simulink library "Completemodels"  (R2014b)
settings: Solver=ode45  StartTime=0.0  StopTime=10.0  RelTol=1e-3
undefined symbols (not defined in the file): X, Y, Z
libraries: sm_lib x26, nesl_utility x24, HexapodLib x18, ServoModel x18, simulink x2
settings Model: Creator=Sebastian  LastModifiedBy=Sebastian

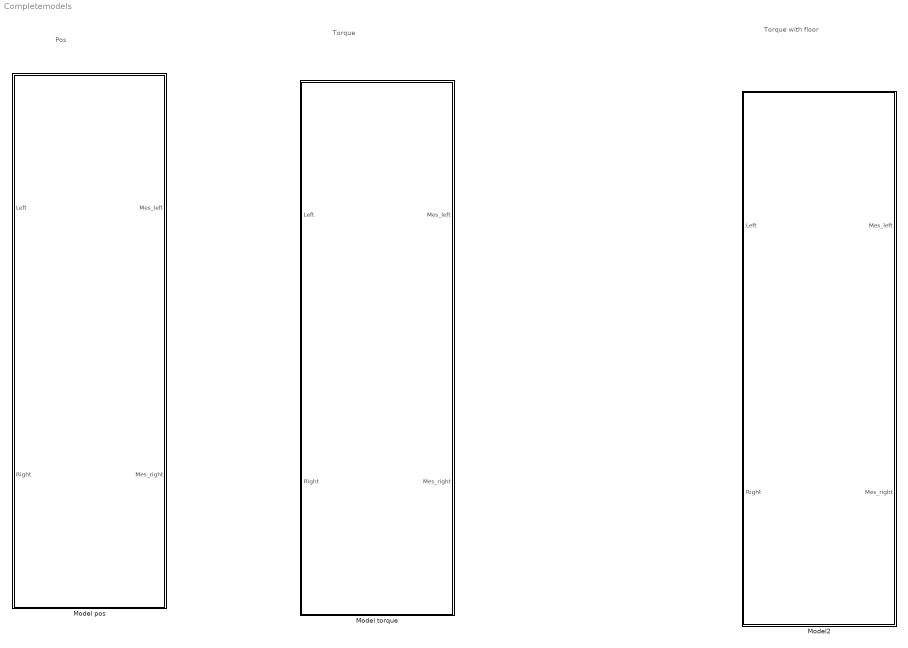
== system Completemodels ==
  note: Pos
  note: Torque
  note: Torque with floor
  Model pos : Subsystem
  Model torque : Subsystem
  Model2 : Subsystem

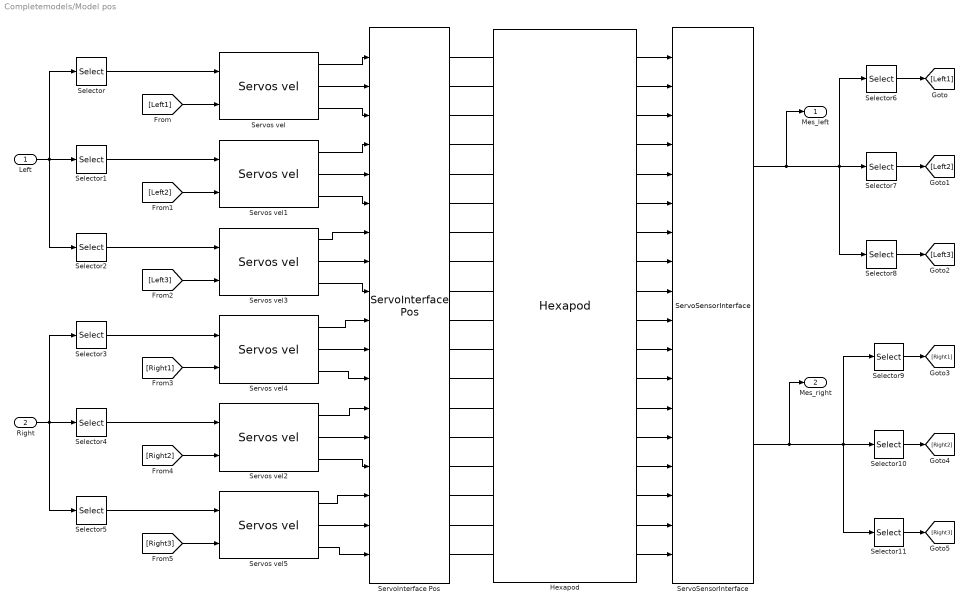
== system Completemodels/Model pos ==
  Left : Inport
  Right : Inport  Port=2
  Hexapod : HexapodLib/Hexapod
  Selector{,3,6,9} (4 alike) : Selector  IndexMode=Zero-based  InputPortWidth=3  Indices=0
  Selector{1,4,7,10} (4 alike) : Selector  IndexMode=Zero-based  InputPortWidth=3
  Selector{2,5,8,11} (4 alike) : Selector  IndexMode=Zero-based  InputPortWidth=3  Indices=2
  ServoInterface Pos : HexapodLib/ServoInterface Pos  Filter_time=0.001
  ServoSensorInterface : HexapodLib/ServoSensorInterface
  Servos vel{,1..5} (6 alike) : ServoModel/Servos vel
  Mes_left : Outport
  Mes_right : Outport  Port=2
  wires:
  Hexapod/9 -> ServoSensorInterface/9
  Servos vel1/1 -> ServoInterface Pos/4
  Hexapod/5 -> ServoSensorInterface/5
  Servos vel5/1 -> ServoInterface Pos/16
  [Right3] -> Servos vel5/2
  Servos vel4/1 -> ServoInterface Pos/10
  Servos vel3/2 -> ServoInterface Pos/8
  Servos vel/2 -> ServoInterface Pos/2
  Servos vel2/3 -> ServoInterface Pos/15
  [Left1] -> Servos vel/2
  [Right1] -> Servos vel4/2
  Servos vel/1 -> ServoInterface Pos/1
  Servos vel/3 -> ServoInterface Pos/3
  Servos vel4/3 -> ServoInterface Pos/12
  Servos vel2/2 -> ServoInterface Pos/14
  [Left3] -> Servos vel3/2
  Servos vel1/3 -> ServoInterface Pos/6
  Servos vel5/3 -> ServoInterface Pos/18
  Servos vel1/2 -> ServoInterface Pos/5
  [Right2] -> Servos vel2/2
  Servos vel3/3 -> ServoInterface Pos/9
  Servos vel4/2 -> ServoInterface Pos/11
  [Left2] -> Servos vel1/2
  Servos vel2/1 -> ServoInterface Pos/13
  Servos vel3/1 -> ServoInterface Pos/7
  Hexapod/10 -> ServoSensorInterface/10
  Hexapod/7 -> ServoSensorInterface/7
  Hexapod/4 -> ServoSensorInterface/4
  Servos vel5/2 -> ServoInterface Pos/17
  Hexapod/8 -> ServoSensorInterface/8
  Hexapod/3 -> ServoSensorInterface/3
  Hexapod/2 -> ServoSensorInterface/2
  Hexapod/1 -> ServoSensorInterface/1
  Hexapod/6 -> ServoSensorInterface/6
  Hexapod/18 -> ServoSensorInterface/18
  Hexapod/17 -> ServoSensorInterface/17
  Hexapod/16 -> ServoSensorInterface/16
  Hexapod/15 -> ServoSensorInterface/15
  Hexapod/14 -> ServoSensorInterface/14
  Hexapod/13 -> ServoSensorInterface/13
  Hexapod/12 -> ServoSensorInterface/12
  Hexapod/11 -> ServoSensorInterface/11
  Left/1 -> Selector2/1, Selector/1, Selector1/1
  Selector1/1 -> Servos vel1/1
  Selector/1 -> Servos vel/1
  Selector2/1 -> Servos vel3/1
  Right/1 -> Selector3/1, Selector5/1, Selector4/1
  Selector4/1 -> Servos vel2/1
  Selector3/1 -> Servos vel4/1
  Selector5/1 -> Servos vel5/1
  ServoSensorInterface/1 -> Selector8/1, Selector6/1, Selector7/1, Mes_left/1
  Selector6/1 -> [Left1]
  Selector7/1 -> [Left2]
  Selector8/1 -> [Left3]
  ServoSensorInterface/2 -> Selector11/1, Selector9/1, Selector10/1, Mes_right/1
  Selector9/1 -> [Right1]
  Selector10/1 -> [Right2]
  Selector11/1 -> [Right3]
  connections:
  Hexapod/LConn7 -- ServoInterface Pos/RConn7
  Hexapod/LConn5 -- ServoInterface Pos/RConn5
  Hexapod/LConn3 -- ServoInterface Pos/RConn3
  Hexapod/LConn16 -- ServoInterface Pos/RConn16
  Hexapod/LConn15 -- ServoInterface Pos/RConn15
  Hexapod/LConn18 -- ServoInterface Pos/RConn18
  Hexapod/LConn14 -- ServoInterface Pos/RConn14
  Hexapod/LConn13 -- ServoInterface Pos/RConn13
  Hexapod/LConn17 -- ServoInterface Pos/RConn17
  Hexapod/LConn11 -- ServoInterface Pos/RConn11
  Hexapod/LConn12 -- ServoInterface Pos/RConn12
  Hexapod/LConn10 -- ServoInterface Pos/RConn10
  Hexapod/LConn8 -- ServoInterface Pos/RConn8
  Hexapod/LConn9 -- ServoInterface Pos/RConn9
  Hexapod/LConn2 -- ServoInterface Pos/RConn2
  Hexapod/LConn4 -- ServoInterface Pos/RConn4
  Hexapod/LConn6 -- ServoInterface Pos/RConn6
  Hexapod/LConn1 -- ServoInterface Pos/RConn1

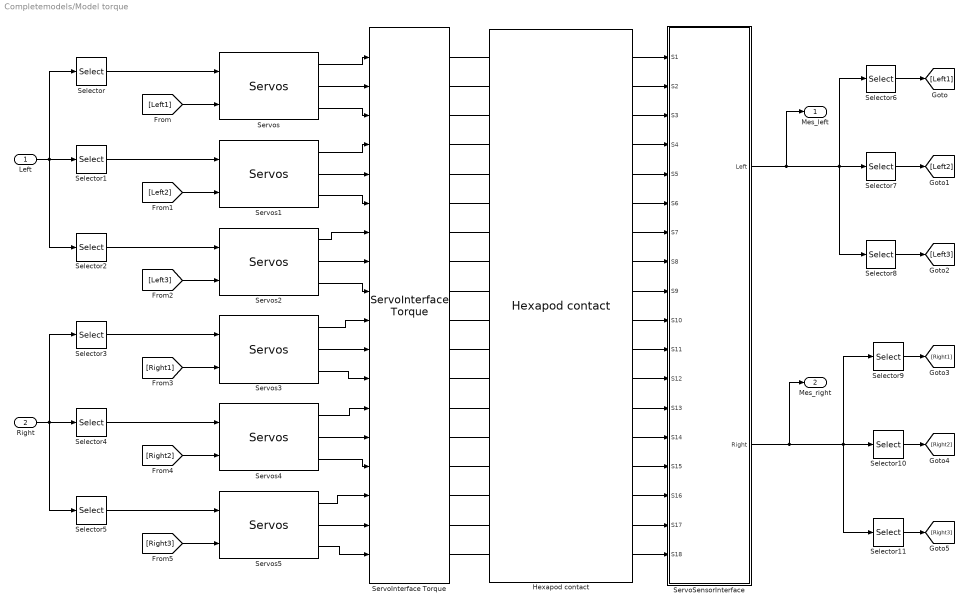
== system Completemodels/Model torque ==
  Left : Inport
  Right : Inport  Port=2
  Hexapod contact : HexapodLib/Hexapod contact
  Selector{,3,6,9} (4 alike) : Selector  IndexMode=Zero-based  InputPortWidth=3  Indices=0
  Selector{1,4,7,10} (4 alike) : Selector  IndexMode=Zero-based  InputPortWidth=3
  Selector{2,5,8,11} (4 alike) : Selector  IndexMode=Zero-based  InputPortWidth=3  Indices=2
  ServoInterface Torque : HexapodLib/ServoInterface Torque
  ServoSensorInterface : Subsystem
  Servos{,1..5} (6 alike) : ServoModel/Servos
  Mes_left : Outport
  Mes_right : Outport  Port=2
  wires:
  Hexapod contact/9 -> ServoSensorInterface/9(S9)
  Servos1/1 -> ServoInterface Torque/4
  Hexapod contact/5 -> ServoSensorInterface/5(S5)
  Servos5/1 -> ServoInterface Torque/16
  [Right3] -> Servos5/2
  Servos3/1 -> ServoInterface Torque/10
  Servos2/2 -> ServoInterface Torque/8
  Servos/2 -> ServoInterface Torque/2
  Servos4/3 -> ServoInterface Torque/15
  [Left1] -> Servos/2
  [Right1] -> Servos3/2
  Servos/1 -> ServoInterface Torque/1
  Servos/3 -> ServoInterface Torque/3
  Servos3/3 -> ServoInterface Torque/12
  Servos4/2 -> ServoInterface Torque/14
  [Left3] -> Servos2/2
  Servos1/3 -> ServoInterface Torque/6
  Servos5/3 -> ServoInterface Torque/18
  Servos1/2 -> ServoInterface Torque/5
  [Right2] -> Servos4/2
  Servos2/3 -> ServoInterface Torque/9
  Servos3/2 -> ServoInterface Torque/11
  [Left2] -> Servos1/2
  Servos4/1 -> ServoInterface Torque/13
  Servos2/1 -> ServoInterface Torque/7
  Hexapod contact/10 -> ServoSensorInterface/10(S10)
  Hexapod contact/7 -> ServoSensorInterface/7(S7)
  Hexapod contact/4 -> ServoSensorInterface/4(S4)
  Servos5/2 -> ServoInterface Torque/17
  Hexapod contact/8 -> ServoSensorInterface/8(S8)
  Hexapod contact/3 -> ServoSensorInterface/3(S3)
  Hexapod contact/2 -> ServoSensorInterface/2(S2)
  Hexapod contact/1 -> ServoSensorInterface/1(S1)
  Hexapod contact/6 -> ServoSensorInterface/6(S6)
  Hexapod contact/18 -> ServoSensorInterface/18(S18)
  Hexapod contact/17 -> ServoSensorInterface/17(S17)
  Hexapod contact/16 -> ServoSensorInterface/16(S16)
  Hexapod contact/15 -> ServoSensorInterface/15(S15)
  Hexapod contact/14 -> ServoSensorInterface/14(S14)
  Hexapod contact/13 -> ServoSensorInterface/13(S13)
  Hexapod contact/12 -> ServoSensorInterface/12(S12)
  Hexapod contact/11 -> ServoSensorInterface/11(S11)
  Left/1 -> Selector2/1, Selector/1, Selector1/1
  Selector1/1 -> Servos1/1
  Selector/1 -> Servos/1
  Selector2/1 -> Servos2/1
  Right/1 -> Selector3/1, Selector5/1, Selector4/1
  Selector4/1 -> Servos4/1
  Selector3/1 -> Servos3/1
  Selector5/1 -> Servos5/1
  ServoSensorInterface/1(Left) -> Selector8/1, Selector6/1, Selector7/1, Mes_left/1
  Selector6/1 -> [Left1]
  Selector7/1 -> [Left2]
  Selector8/1 -> [Left3]
  ServoSensorInterface/2(Right) -> Selector11/1, Selector9/1, Selector10/1, Mes_right/1
  Selector9/1 -> [Right1]
  Selector10/1 -> [Right2]
  Selector11/1 -> [Right3]
  connections:
  Hexapod contact/LConn7 -- ServoInterface Torque/RConn7
  Hexapod contact/LConn5 -- ServoInterface Torque/RConn5
  Hexapod contact/LConn3 -- ServoInterface Torque/RConn3
  Hexapod contact/LConn16 -- ServoInterface Torque/RConn16
  Hexapod contact/LConn15 -- ServoInterface Torque/RConn15
  Hexapod contact/LConn18 -- ServoInterface Torque/RConn18
  Hexapod contact/LConn14 -- ServoInterface Torque/RConn14
  Hexapod contact/LConn13 -- ServoInterface Torque/RConn13
  Hexapod contact/LConn17 -- ServoInterface Torque/RConn17
  Hexapod contact/LConn11 -- ServoInterface Torque/RConn11
  Hexapod contact/LConn12 -- ServoInterface Torque/RConn12
  Hexapod contact/LConn10 -- ServoInterface Torque/RConn10
  Hexapod contact/LConn8 -- ServoInterface Torque/RConn8
  Hexapod contact/LConn9 -- ServoInterface Torque/RConn9
  Hexapod contact/LConn2 -- ServoInterface Torque/RConn2
  Hexapod contact/LConn4 -- ServoInterface Torque/RConn4
  Hexapod contact/LConn6 -- ServoInterface Torque/RConn6
  Hexapod contact/LConn1 -- ServoInterface Torque/RConn1

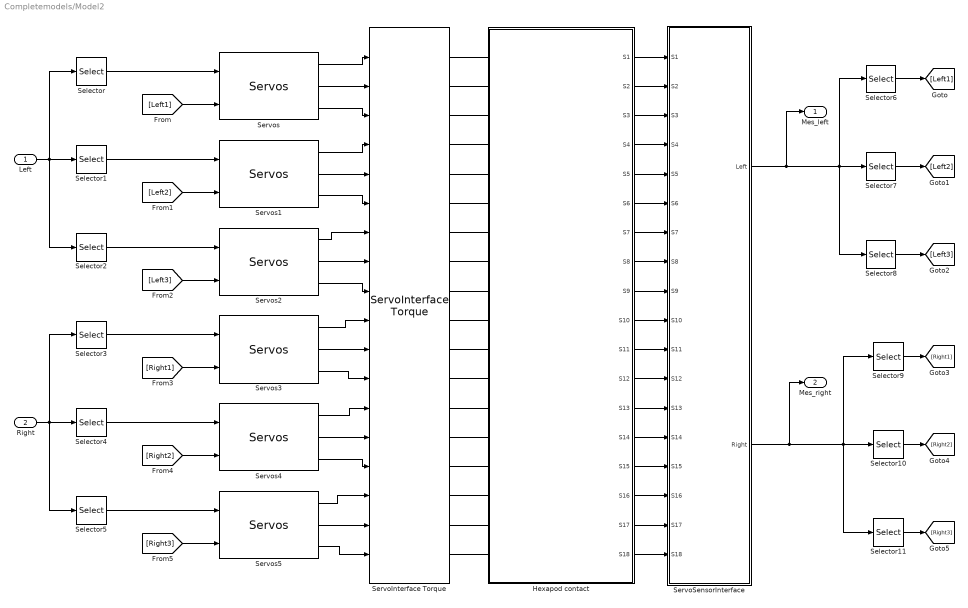
== system Completemodels/Model2 ==
  Left : Inport
  Right : Inport  Port=2
  Hexapod contact : Subsystem
  Selector{,3,6,9} (4 alike) : Selector  IndexMode=Zero-based  InputPortWidth=3  Indices=0
  Selector{1,4,7,10} (4 alike) : Selector  IndexMode=Zero-based  InputPortWidth=3
  Selector{2,5,8,11} (4 alike) : Selector  IndexMode=Zero-based  InputPortWidth=3  Indices=2
  ServoInterface Torque : HexapodLib/ServoInterface Torque
  ServoSensorInterface : Subsystem
  Servos{,1..5} (6 alike) : ServoModel/Servos
  Mes_left : Outport
  Mes_right : Outport  Port=2
  wires:
  Hexapod contact/9(S9) -> ServoSensorInterface/9(S9)
  Servos1/1 -> ServoInterface Torque/4
  Hexapod contact/5(S5) -> ServoSensorInterface/5(S5)
  Servos5/1 -> ServoInterface Torque/16
  [Right3] -> Servos5/2
  Servos3/1 -> ServoInterface Torque/10
  Servos2/2 -> ServoInterface Torque/8
  Servos/2 -> ServoInterface Torque/2
  Servos4/3 -> ServoInterface Torque/15
  [Left1] -> Servos/2
  [Right1] -> Servos3/2
  Servos/1 -> ServoInterface Torque/1
  Servos/3 -> ServoInterface Torque/3
  Servos3/3 -> ServoInterface Torque/12
  Servos4/2 -> ServoInterface Torque/14
  [Left3] -> Servos2/2
  Servos1/3 -> ServoInterface Torque/6
  Servos5/3 -> ServoInterface Torque/18
  Servos1/2 -> ServoInterface Torque/5
  [Right2] -> Servos4/2
  Servos2/3 -> ServoInterface Torque/9
  Servos3/2 -> ServoInterface Torque/11
  [Left2] -> Servos1/2
  Servos4/1 -> ServoInterface Torque/13
  Servos2/1 -> ServoInterface Torque/7
  Hexapod contact/10(S10) -> ServoSensorInterface/10(S10)
  Hexapod contact/7(S7) -> ServoSensorInterface/7(S7)
  Hexapod contact/4(S4) -> ServoSensorInterface/4(S4)
  Servos5/2 -> ServoInterface Torque/17
  Hexapod contact/8(S8) -> ServoSensorInterface/8(S8)
  Hexapod contact/3(S3) -> ServoSensorInterface/3(S3)
  Hexapod contact/2(S2) -> ServoSensorInterface/2(S2)
  Hexapod contact/1(S1) -> ServoSensorInterface/1(S1)
  Hexapod contact/6(S6) -> ServoSensorInterface/6(S6)
  Hexapod contact/18(S18) -> ServoSensorInterface/18(S18)
  Hexapod contact/17(S17) -> ServoSensorInterface/17(S17)
  Hexapod contact/16(S16) -> ServoSensorInterface/16(S16)
  Hexapod contact/15(S15) -> ServoSensorInterface/15(S15)
  Hexapod contact/14(S14) -> ServoSensorInterface/14(S14)
  Hexapod contact/13(S13) -> ServoSensorInterface/13(S13)
  Hexapod contact/12(S12) -> ServoSensorInterface/12(S12)
  Hexapod contact/11(S11) -> ServoSensorInterface/11(S11)
  Left/1 -> Selector2/1, Selector/1, Selector1/1
  Selector1/1 -> Servos1/1
  Selector/1 -> Servos/1
  Selector2/1 -> Servos2/1
  Right/1 -> Selector3/1, Selector5/1, Selector4/1
  Selector4/1 -> Servos4/1
  Selector3/1 -> Servos3/1
  Selector5/1 -> Servos5/1
  ServoSensorInterface/1(Left) -> Selector8/1, Selector6/1, Selector7/1, Mes_left/1
  Selector6/1 -> [Left1]
  Selector7/1 -> [Left2]
  Selector8/1 -> [Left3]
  ServoSensorInterface/2(Right) -> Selector11/1, Selector9/1, Selector10/1, Mes_right/1
  Selector9/1 -> [Right1]
  Selector10/1 -> [Right2]
  Selector11/1 -> [Right3]
  connections:
  Hexapod contact/LConn7 -- ServoInterface Torque/RConn7
  Hexapod contact/LConn5 -- ServoInterface Torque/RConn5
  Hexapod contact/LConn3 -- ServoInterface Torque/RConn3
  Hexapod contact/LConn16 -- ServoInterface Torque/RConn16
  Hexapod contact/LConn15 -- ServoInterface Torque/RConn15
  Hexapod contact/LConn18 -- ServoInterface Torque/RConn18
  Hexapod contact/LConn14 -- ServoInterface Torque/RConn14
  Hexapod contact/LConn13 -- ServoInterface Torque/RConn13
  Hexapod contact/LConn17 -- ServoInterface Torque/RConn17
  Hexapod contact/LConn11 -- ServoInterface Torque/RConn11
  Hexapod contact/LConn12 -- ServoInterface Torque/RConn12
  Hexapod contact/LConn10 -- ServoInterface Torque/RConn10
  Hexapod contact/LConn8 -- ServoInterface Torque/RConn8
  Hexapod contact/LConn9 -- ServoInterface Torque/RConn9
  Hexapod contact/LConn2 -- ServoInterface Torque/RConn2
  Hexapod contact/LConn4 -- ServoInterface Torque/RConn4
  Hexapod contact/LConn6 -- ServoInterface Torque/RConn6
  Hexapod contact/LConn1 -- ServoInterface Torque/RConn1

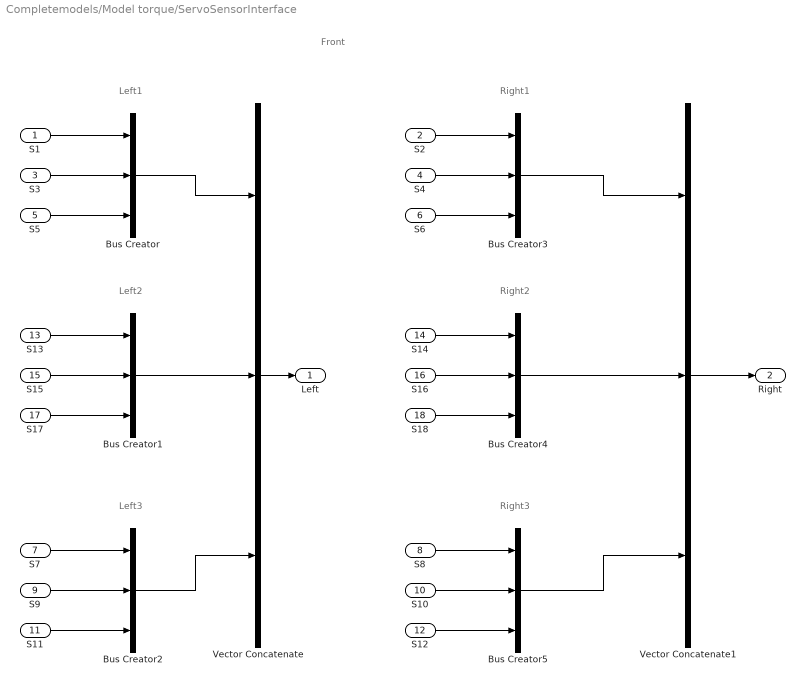
== system Completemodels/Model torque/ServoSensorInterface ==
  note: Front
  note: Left1
  note: Left2
  note: Left3
  note: Right1
  note: Right2
  note: Right3
  S1 : Inport
  S2 : Inport  Port=2
  S3 : Inport  Port=3
  S4 : Inport  Port=4
  S5 : Inport  Port=5
  S6 : Inport  Port=6
  S7 : Inport  Port=7
  S8 : Inport  Port=8
  S9 : Inport  Port=9
  S10 : Inport  Port=10
  S11 : Inport  Port=11
  S12 : Inport  Port=12
  S13 : Inport  Port=13
  S14 : Inport  Port=14
  S15 : Inport  Port=15
  S16 : Inport  Port=16
  S17 : Inport  Port=17
  S18 : Inport  Port=18
  Bus Creator{,1..5} (6 alike) : BusCreator  Inputs=3  OutDataTypeStr=Bus: Leg_mes  NonVirtualBus=on
  Vector Concatenate : Concatenate  NumInputs=3  ConcatenateDimension=2
  Vector Concatenate1 : Concatenate  NumInputs=3  ConcatenateDimension=2
  Left : Outport
  Right : Outport  Port=2
  wires:
  Bus Creator1/1 -> Vector Concatenate/2
  Bus Creator2/1 -> Vector Concatenate/3
  Bus Creator3/1 -> Vector Concatenate1/1
  Bus Creator5/1 -> Vector Concatenate1/3
  S2/1 -> Bus Creator3/1
  S4/1 -> Bus Creator3/2
  S6/1 -> Bus Creator3/3
  S14/1 -> Bus Creator4/1
  S16/1 -> Bus Creator4/2
  S18/1 -> Bus Creator4/3
  S8/1 -> Bus Creator5/1
  S10/1 -> Bus Creator5/2
  S12/1 -> Bus Creator5/3
  S1/1 -> Bus Creator/1
  S3/1 -> Bus Creator/2
  S5/1 -> Bus Creator/3
  S13/1 -> Bus Creator1/1
  S15/1 -> Bus Creator1/2
  S17/1 -> Bus Creator1/3
  S7/1 -> Bus Creator2/1
  S9/1 -> Bus Creator2/2
  S11/1 -> Bus Creator2/3
  Bus Creator/1 -> Vector Concatenate/1
  Vector Concatenate/1 -> Left/1
  Bus Creator4/1 -> Vector Concatenate1/2
  Vector Concatenate1/1 -> Right/1

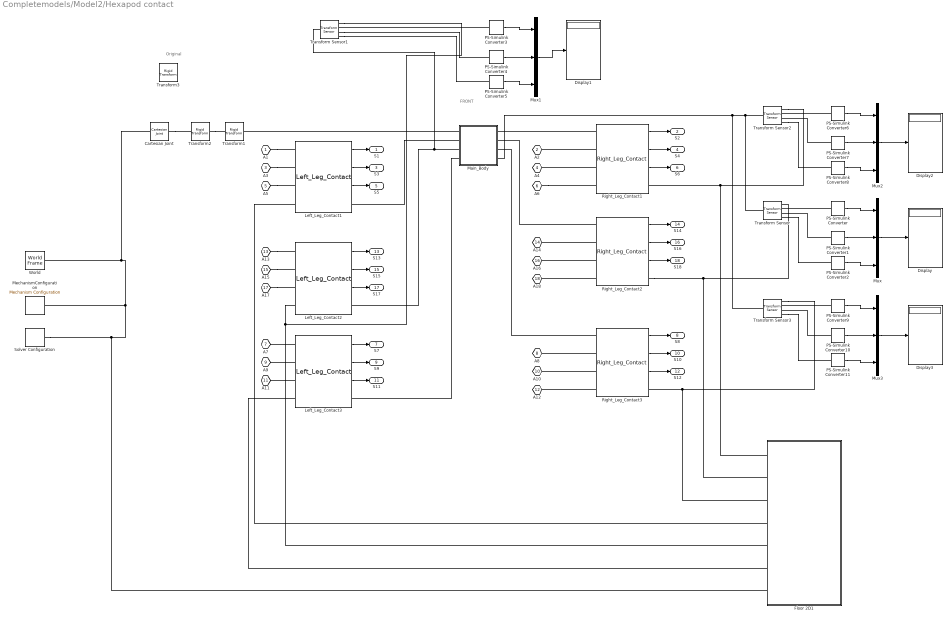
== system Completemodels/Model2/Hexapod contact ==
  note: Original
  note: FRONT
  Cartesian Joint : sm_lib/Joints/Cartesian Joint  SenseConstraintForce=off  SenseConstraintForceX=off  SenseConstraintForceY=off  SenseConstraintForceZ=off  SenseConstraintTorque=off  SenseConstraintTorqueX=off  SenseConstraintTorqueY=off  SenseConstraintTorqueZ=off  SenseTotalForce=off  SenseTotalForceX=off  SenseTotalForceY=off  SenseTotalForceZ=off  SenseTotalTorque=off  SenseTotalTorqueX=off  SenseTotalTorqueY=off  SenseTotalTorqueZ=off  CompositeWrenchDir=FollowerOnBase  CompositeWrenchFrame=BaseFrame  PxEquilibriumPosition=0  PxEquilibriumPositionUnits=m  PxSpringStiffness=0  PxSpringStiffnessUnits=N/m  PxDampingCoefficient=0  PxDampingCoefficientUnits=N/(m/s)  PxTorqueActuationMode=NoTorque  PxMotionActuationMode=ComputedMotion  PxSensePosition=off  PxSenseVelocity=off  PxSenseAcceleration=off  PxSenseTorqueForce=off  PxPositionTargetValue=0  PxPositionTargetValueUnits=m  PxPositionTargetSpecify=off  PxPositionTargetPriority=High  PxVelocityTargetValue=0  PxVelocityTargetValueUnits=m/s  PxVelocityTargetSpecify=off  PxVelocityTargetPriority=High  PyEquilibriumPosition=0  PyEquilibriumPositionUnits=m  PySpringStiffness=0  PySpringStiffnessUnits=N/m  PyDampingCoefficient=0  PyDampingCoefficientUnits=N/(m/s)  PyTorqueActuationMode=NoTorque  PyMotionActuationMode=ComputedMotion  PySensePosition=off  PySenseVelocity=off  PySenseAcceleration=off  PySenseTorqueForce=off  PyPositionTargetValue=0  PyPositionTargetValueUnits=m  PyPositionTargetSpecify=off  PyPositionTargetPriority=High  PyVelocityTargetValue=0  PyVelocityTargetValueUnits=m/s  PyVelocityTargetSpecify=off  PyVelocityTargetPriority=High  PzEquilibriumPosition=0  PzEquilibriumPositionUnits=m  PzSpringStiffness=0  PzSpringStiffnessUnits=N/m  PzDampingCoefficient=0  PzDampingCoefficientUnits=N/(m/s)  PzTorqueActuationMode=NoTorque  PzMotionActuationMode=ComputedMotion  PzSensePosition=off  PzSenseVelocity=off  PzSenseAcceleration=off  PzSenseTorqueForce=off  PzPositionTargetValue=0  PzPositionTargetValueUnits=m  PzPositionTargetSpecify=off  PzPositionTargetPriority=High  PzVelocityTargetValue=0  PzVelocityTargetValueUnits=m/s  PzVelocityTargetSpecify=off  PzVelocityTargetPriority=High  BlockFunction=simmechanics.library.joints.cartesian_joint
  Display{,1..3} (4 alike) : Display
  Floor 2D1 : Subsystem
  Left_Leg_Contact1 : HexapodLib/Left_Leg_Contact  SystemSampleTime=-1
  Left_Leg_Contact2 : HexapodLib/Left_Leg_Contact  SystemSampleTime=-1
  Left_Leg_Contact3 : HexapodLib/Left_Leg_Contact  SystemSampleTime=-1
  Main_Body : Subsystem  AncestorBlock=HexapodLib/Main_Body
  MechanismConfiguration : sm_lib/Utilities/Mechanism Configuration  UniformGravity=Constant  GravityVector=[0 0 -9.82]  GravityUnits=m/s^2  LinearizationDelta=0.001  BlockFunction=simmechanics.library.utilities.mechanism_configuration
  Mux{,1..3} (4 alike) : Mux  Inputs=3
  PS-Simulink Converter{,1..11} (12 alike) : nesl_utility/PS-Simulink Converter  PhysicalDomain=network_engine_domain  SubClassName=ps_output  LeftPortType=input  RightPortType=output  PseudoPeriodic=off  Frequencies=[]  Unit=mm  AffineConversion=off
  Right_Leg_Contact1 : HexapodLib/Right_Leg_Contact  SystemSampleTime=-1
  Right_Leg_Contact2 : HexapodLib/Right_Leg_Contact  SystemSampleTime=-1
  Right_Leg_Contact3 : HexapodLib/Right_Leg_Contact  SystemSampleTime=-1
  Solver Configuration : nesl_utility/Solver Configuration  PhysicalDomain=network_engine_domain  SubClassName=solver  LeftPortType=input  RightPortType=generic  Accelerate=off  Tones=[]  Harmonics=[]  SimulateNoise=off  Profile=off  UseLocalSampling=off  EnableSwitchedLinearOptims=on  FrequencyDomain=off  UseCCode=off  RelTol=0.001  AbsTol=1e-06  MinStep=1e-09  ToWorkspace=off  DoDC=off  ResidualTolerance=1e-09  UseLocalSolver=off  LocalSolverChoice=NE_BACKWARD_EULER_ADVANCER  LocalSolverSampleTime=0.001  DoFixedCost=off  MaxNonlinIter=3  MaxModeIter=2  LinearAlgebra=Sparse  DelaysMemoryBudget=1024  AutomaticFiltering=on  FilteringTimeConstant=0.001
  Transform Sensor{,1..3} (4 alike) : sm_lib/Frames and Transforms/Transform Sensor  MeasurementFrame=Base  SenseAngle=off  SenseAxis=off  SenseAngle1=off  SenseAngle2=off  SenseAngle3=off  SenseQ=off  SenseR=off  SenseOmegaX=off  SenseOmegaY=off  SenseOmegaZ=off  SenseOmega1=off  SenseOmega2=off  SenseOmega3=off  SenseQDot=off  SenseRDot=off  SenseAlphaX=off  SenseAlphaY=off  SenseAlphaZ=off  SenseAlpha1=off  SenseAlpha2=off  SenseAlpha3=off  SenseQDDot=off  SenseRDDot=off  SenseX=on  SenseY=on  SenseZ=on  SenseRad=off  SenseAzim=off  SenseDist=off  SenseInc=off  SenseXDot=off  SenseYDot=off  SenseZDot=off  SenseRadDot=off  SenseAzimDot=off  SenseDistDot=off  SenseIncDot=off  SenseXDDot=off  SenseYDDot=off  SenseZDDot=off  SenseRadDDot=off  SenseAzimDDot=off  SenseDistDDot=off  SenseIncDDot=off  BlockFunction=simmechanics.library.frames_transforms.transform_sensor
  Transform1 : sm_lib/Frames and Transforms/Rigid Transform  TranslationMethod=None  TranslationLengthUnit=cm  TranslationStandardAxis=+Z  TranslationStandardOffset=0  TranslationCartesianOffset=[0 0 93]  TranslationROffset=0  TranslationROffsetUnits=m  TranslationZOffset=0  TranslationZOffsetUnits=m  TranslationThetaOffset=0  TranslationThetaOffsetUnits=deg  RotationMethod=StandardAxis  RotationAngleUnits=deg  RotationStandardAxis=+Z  RotationAngle=180  RotationArbitraryAxis=[0 0 0]  FollAlignAxisA=+X  BaseAlignAxisA=+Y  FollAlignAxisB=+Y  BaseAlignAxisB=+Z  RotationMatrix=[1 0 0; 0 1 0; 0 0 1]  BlockFunction=simmechanics.library.frames_transforms.rigid_transform
  Transform2 : sm_lib/Frames and Transforms/Rigid Transform  TranslationMethod=Cartesian  TranslationLengthUnit=cm  TranslationStandardAxis=+Z  TranslationStandardOffset=0  TranslationCartesianOffset=[0 0 30]  TranslationROffset=0  TranslationROffsetUnits=m  TranslationZOffset=0  TranslationZOffsetUnits=m  TranslationThetaOffset=0  TranslationThetaOffsetUnits=deg  RotationMethod=None  RotationAngleUnits=deg  RotationStandardAxis=+Z  RotationAngle=180  RotationArbitraryAxis=[0 0 0]  FollAlignAxisA=+X  BaseAlignAxisA=+Y  FollAlignAxisB=+Y  BaseAlignAxisB=+Z  RotationMatrix=[1 0 0; 0 1 0; 0 0 1]  BlockFunction=simmechanics.library.frames_transforms.rigid_transform
  Transform3 : sm_lib/Frames and Transforms/Rigid Transform  TranslationMethod=Cartesian  TranslationLengthUnit=cm  TranslationStandardAxis=+Z  TranslationStandardOffset=0  TranslationCartesianOffset=[0 0 93]  TranslationROffset=0  TranslationROffsetUnits=m  TranslationZOffset=0  TranslationZOffsetUnits=m  TranslationThetaOffset=0  TranslationThetaOffsetUnits=deg  RotationMethod=StandardAxis  RotationAngleUnits=deg  RotationStandardAxis=+Z  RotationAngle=180  RotationArbitraryAxis=[0 0 0]  FollAlignAxisA=+X  BaseAlignAxisA=+Y  FollAlignAxisB=+Y  BaseAlignAxisB=+Z  RotationMatrix=[1 0 0; 0 1 0; 0 0 1]  BlockFunction=simmechanics.library.frames_transforms.rigid_transform
  World : sm_lib/Frames and Transforms/World Frame  BlockFunction=simmechanics.library.frames_transforms.world_frame
  A1 : PMIOPort  Port=1  Side=Left
  A2 : PMIOPort  Port=2  Side=Left
  A3 : PMIOPort  Port=3  Side=Left
  A4 : PMIOPort  Port=4  Side=Left
  A5 : PMIOPort  Port=5  Side=Left
  A6 : PMIOPort  Port=6  Side=Left
  A7 : PMIOPort  Port=7  Side=Left
  A8 : PMIOPort  Port=8  Side=Left
  A9 : PMIOPort  Port=9  Side=Left
  A10 : PMIOPort  Port=10  Side=Left
  A11 : PMIOPort  Port=11  Side=Left
  A12 : PMIOPort  Port=12  Side=Left
  A13 : PMIOPort  Port=13  Side=Left
  A14 : PMIOPort  Port=14  Side=Left
  A15 : PMIOPort  Port=15  Side=Left
  A16 : PMIOPort  Port=16  Side=Left
  A17 : PMIOPort  Port=17  Side=Left
  A18 : PMIOPort  Port=18  Side=Left
  S1 : Outport
  S2 : Outport  Port=2
  S3 : Outport  Port=3
  S4 : Outport  Port=4
  S5 : Outport  Port=5
  S6 : Outport  Port=6
  S7 : Outport  Port=7
  S8 : Outport  Port=8
  S9 : Outport  Port=9
  S10 : Outport  Port=10
  S11 : Outport  Port=11
  S12 : Outport  Port=12
  S13 : Outport  Port=13
  S14 : Outport  Port=14
  S15 : Outport  Port=15
  S16 : Outport  Port=16
  S17 : Outport  Port=17
  S18 : Outport  Port=18
  wires:
  Mux1/1 -> Display1/1
  PS-Simulink Converter5/1 -> Mux1/3
  PS-Simulink Converter4/1 -> Mux1/2
  PS-Simulink Converter3/1 -> Mux1/1
  Mux/1 -> Display/1
  PS-Simulink Converter2/1 -> Mux/3
  PS-Simulink Converter1/1 -> Mux/2
  PS-Simulink Converter/1 -> Mux/1
  Right_Leg_Contact2/3 -> S18/1
  Right_Leg_Contact2/2 -> S16/1
  Right_Leg_Contact2/1 -> S14/1
  Right_Leg_Contact3/3 -> S12/1
  Right_Leg_Contact3/2 -> S10/1
  Right_Leg_Contact3/1 -> S8/1
  Right_Leg_Contact1/3 -> S6/1
  Right_Leg_Contact1/2 -> S4/1
  Right_Leg_Contact1/1 -> S2/1
  Left_Leg_Contact1/2 -> S3/1
  Left_Leg_Contact1/1 -> S1/1
  Left_Leg_Contact1/3 -> S5/1
  Left_Leg_Contact2/1 -> S13/1
  Left_Leg_Contact2/2 -> S15/1
  Left_Leg_Contact2/3 -> S17/1
  Left_Leg_Contact3/1 -> S7/1
  Left_Leg_Contact3/2 -> S9/1
  Left_Leg_Contact3/3 -> S11/1
  Mux2/1 -> Display2/1
  PS-Simulink Converter8/1 -> Mux2/3
  PS-Simulink Converter7/1 -> Mux2/2
  PS-Simulink Converter6/1 -> Mux2/1
  Mux3/1 -> Display3/1
  PS-Simulink Converter11/1 -> Mux3/3
  PS-Simulink Converter10/1 -> Mux3/2
  PS-Simulink Converter9/1 -> Mux3/1
  connections:
  Transform Sensor1/RConn3 -- PS-Simulink Converter4/LConn1
  PS-Simulink Converter3/LConn1 -- Transform Sensor1/RConn2
  Transform Sensor1/RConn4 -- PS-Simulink Converter5/LConn1
  Transform Sensor/RConn4 -- PS-Simulink Converter2/LConn1
  PS-Simulink Converter1/LConn1 -- Transform Sensor/RConn3
  PS-Simulink Converter/LConn1 -- Transform Sensor/RConn2
  Right_Leg_Contact2/RConn1 -- Floor 2D1/LConn2 -- Transform Sensor/RConn1
  Main_Body/LConn4 -- Left_Leg_Contact3/RConn1
  Left_Leg_Contact2/RConn1 -- Transform Sensor1/LConn1 -- Main_Body/LConn3
  Main_Body/LConn2 -- Left_Leg_Contact1/RConn1
  Transform Sensor1/RConn1 -- Left_Leg_Contact2/LConn4 -- Floor 2D1/LConn5
  A6/RConn1 -- Right_Leg_Contact1/LConn4
  Right_Leg_Contact2/LConn4 -- A18/RConn1
  Right_Leg_Contact3/LConn4 -- A12/RConn1
  Right_Leg_Contact1/LConn3 -- A4/RConn1
  Right_Leg_Contact2/LConn1 -- Main_Body/RConn2
  Right_Leg_Contact1/LConn2 -- A2/RConn1
  Right_Leg_Contact1/LConn1 -- Main_Body/RConn1
  Right_Leg_Contact3/LConn2 -- A8/RConn1
  Right_Leg_Contact3/LConn3 -- A10/RConn1
  Right_Leg_Contact2/LConn2 -- A14/RConn1
  Right_Leg_Contact2/LConn3 -- A16/RConn1
  Transform Sensor2/RConn1 -- Floor 2D1/LConn1 -- Right_Leg_Contact1/RConn1
  Transform Sensor3/RConn1 -- Floor 2D1/LConn3 -- Right_Leg_Contact3/RConn1
  A1/RConn1 -- Left_Leg_Contact1/LConn1
  A3/RConn1 -- Left_Leg_Contact1/LConn2
  A5/RConn1 -- Left_Leg_Contact1/LConn3
  A13/RConn1 -- Left_Leg_Contact2/LConn1
  A15/RConn1 -- Left_Leg_Contact2/LConn2
  A17/RConn1 -- Left_Leg_Contact2/LConn3
  Left_Leg_Contact3/LConn1 -- A7/RConn1
  Left_Leg_Contact3/LConn2 -- A9/RConn1
  Left_Leg_Contact3/LConn3 -- A11/RConn1
  PS-Simulink Converter6/LConn1 -- Transform Sensor2/RConn2
  Transform Sensor2/RConn4 -- PS-Simulink Converter8/LConn1
  PS-Simulink Converter7/LConn1 -- Transform Sensor2/RConn3
  Transform Sensor3/RConn4 -- PS-Simulink Converter11/LConn1
  PS-Simulink Converter9/LConn1 -- Transform Sensor3/RConn2
  PS-Simulink Converter10/LConn1 -- Transform Sensor3/RConn3
  Transform Sensor2/LConn1 -- Transform Sensor/LConn1 -- Transform Sensor3/LConn1 -- Main_Body/RConn4
  Right_Leg_Contact3/LConn1 -- Main_Body/RConn3
  Floor 2D1/LConn4 -- Left_Leg_Contact1/LConn4
  Floor 2D1/LConn6 -- Left_Leg_Contact3/LConn4
  Solver Configuration/RConn1 -- Floor 2D1/LConn7 -- MechanismConfiguration/RConn1 -- Cartesian Joint/LConn1 -- World/RConn1
  Transform2/RConn1 -- Transform1/LConn1
  Main_Body/LConn1 -- Transform1/RConn1
  Cartesian Joint/RConn1 -- Transform2/LConn1

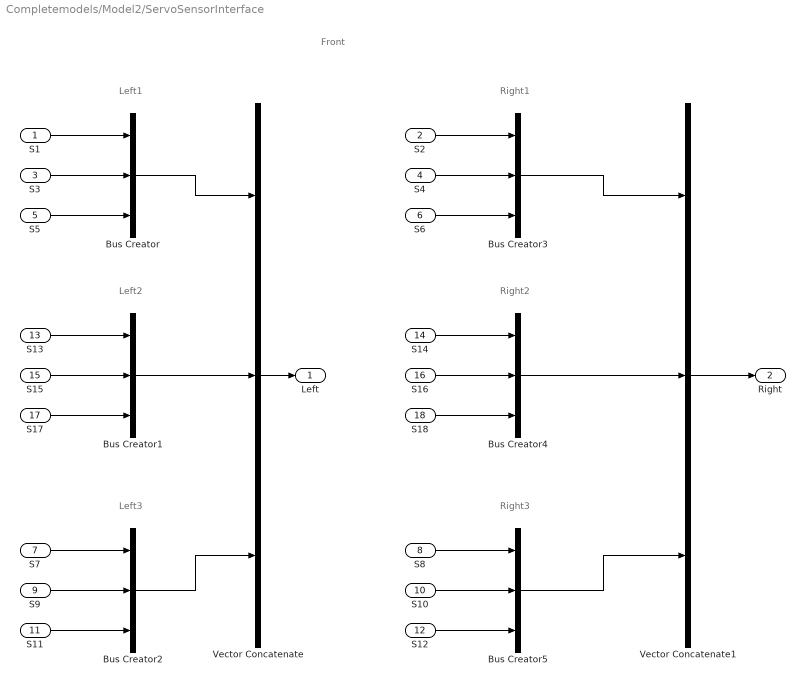
== system Completemodels/Model2/ServoSensorInterface ==
  note: Front
  note: Left1
  note: Left2
  note: Left3
  note: Right1
  note: Right2
  note: Right3
  S1 : Inport
  S2 : Inport  Port=2
  S3 : Inport  Port=3
  S4 : Inport  Port=4
  S5 : Inport  Port=5
  S6 : Inport  Port=6
  S7 : Inport  Port=7
  S8 : Inport  Port=8
  S9 : Inport  Port=9
  S10 : Inport  Port=10
  S11 : Inport  Port=11
  S12 : Inport  Port=12
  S13 : Inport  Port=13
  S14 : Inport  Port=14
  S15 : Inport  Port=15
  S16 : Inport  Port=16
  S17 : Inport  Port=17
  S18 : Inport  Port=18
  Bus Creator{,1..5} (6 alike) : BusCreator  Inputs=3  OutDataTypeStr=Bus: Leg_mes  NonVirtualBus=on
  Vector Concatenate : Concatenate  NumInputs=3  ConcatenateDimension=2
  Vector Concatenate1 : Concatenate  NumInputs=3  ConcatenateDimension=2
  Left : Outport
  Right : Outport  Port=2
  wires:
  Bus Creator1/1 -> Vector Concatenate/2
  Bus Creator2/1 -> Vector Concatenate/3
  Bus Creator3/1 -> Vector Concatenate1/1
  Bus Creator5/1 -> Vector Concatenate1/3
  S2/1 -> Bus Creator3/1
  S4/1 -> Bus Creator3/2
  S6/1 -> Bus Creator3/3
  S14/1 -> Bus Creator4/1
  S16/1 -> Bus Creator4/2
  S18/1 -> Bus Creator4/3
  S8/1 -> Bus Creator5/1
  S10/1 -> Bus Creator5/2
  S12/1 -> Bus Creator5/3
  S1/1 -> Bus Creator/1
  S3/1 -> Bus Creator/2
  S5/1 -> Bus Creator/3
  S13/1 -> Bus Creator1/1
  S15/1 -> Bus Creator1/2
  S17/1 -> Bus Creator1/3
  S7/1 -> Bus Creator2/1
  S9/1 -> Bus Creator2/2
  S11/1 -> Bus Creator2/3
  Bus Creator/1 -> Vector Concatenate/1
  Vector Concatenate/1 -> Left/1
  Bus Creator4/1 -> Vector Concatenate1/2
  Vector Concatenate1/1 -> Right/1

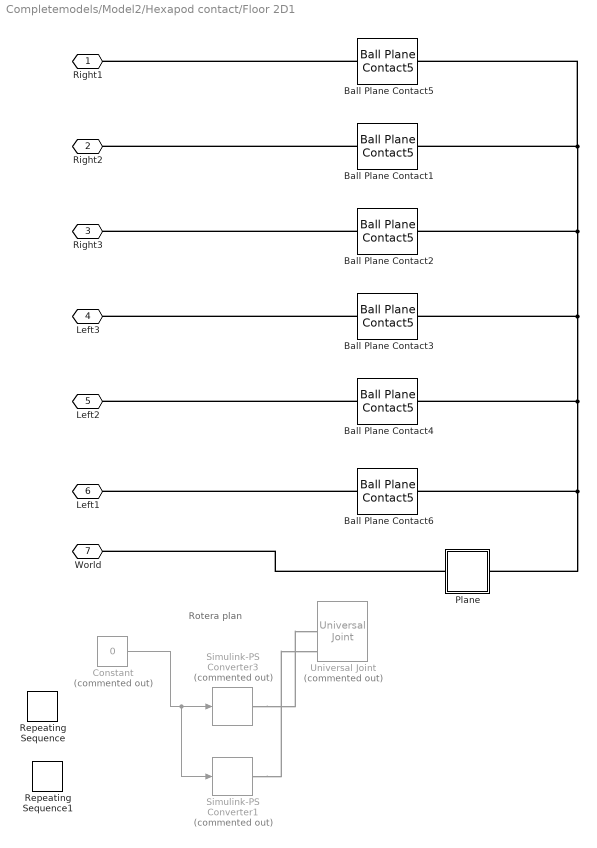
== system Completemodels/Model2/Hexapod contact/Floor 2D1 ==
  note: Rotera plan
  Ball Plane Contact{1..6} (6 alike) : HexapodLib/Ball Plane  Contact5  pz0=zinit  rsph=sprad  hpla=[2.5 2.5 0.05]  Kpen=100000  Dpen=100  mustat=1  vthr=fvel
  Constant : Constant  Commented=on  Value=0
  Plane : Subsystem
  Repeating Sequence : simulink/Sources/Repeating Sequence  rep_seq_t=[0 2 2.5 4 5 7.7 8.2 20]  rep_seq_y=-0.03*[0 0 1 1 -1 -1 0 0]
  Repeating Sequence1 : simulink/Sources/Repeating Sequence  rep_seq_t=[0 7 7.5 9 10 13 13.5 20]  rep_seq_y=-0.03*[0 0 1 1 -1 -1 0 0]
  Simulink-PS Converter1 : nesl_utility/Simulink-PS Converter  Commented=on  PhysicalDomain=network_engine_domain  SubClassName=ps_input  LeftPortType=input  RightPortType=output  PseudoPeriodic=off  Frequencies=[]  NoiseDistribution=none  NoiseParameters=[]  Unit=1  AffineConversion=off  InputFiltering=on  SimscapeFilterOrder=2  InputFilterTimeConstant=0.1  UdotUserProvided=2
  Simulink-PS Converter3 : nesl_utility/Simulink-PS Converter  Commented=on  PhysicalDomain=network_engine_domain  SubClassName=ps_input  LeftPortType=input  RightPortType=output  PseudoPeriodic=off  Frequencies=[]  NoiseDistribution=none  NoiseParameters=[]  Unit=1  AffineConversion=off  InputFiltering=on  SimscapeFilterOrder=2  InputFilterTimeConstant=0.1  UdotUserProvided=2
  Universal Joint : sm_lib/Joints/Universal Joint  Commented=on  SenseConstraintForce=off  SenseConstraintForceX=off  SenseConstraintForceY=off  SenseConstraintForceZ=off  SenseConstraintTorque=off  SenseConstraintTorqueX=off  SenseConstraintTorqueY=off  SenseConstraintTorqueZ=off  SenseTotalForce=off  SenseTotalForceX=off  SenseTotalForceY=off  SenseTotalForceZ=off  SenseTotalTorque=off  SenseTotalTorqueX=off  SenseTotalTorqueY=off  SenseTotalTorqueZ=off  CompositeWrenchDir=FollowerOnBase  CompositeWrenchFrame=BaseFrame  RxEquilibriumPosition=0  RxEquilibriumPositionUnits=deg  RxSpringStiffness=0  RxSpringStiffnessUnits=N*m/deg  RxDampingCoefficient=0  RxDampingCoefficientUnits=N*m/(deg/s)  RxTorqueActuationMode=ComputedTorque  RxMotionActuationMode=InputMotion  RxSensePosition=off  RxSenseVelocity=off  RxSenseAcceleration=off  RxSenseTorqueForce=off  RxPositionTargetValue=0  RxPositionTargetValueUnits=deg  RxPositionTargetSpecify=off  RxPositionTargetPriority=High  RxVelocityTargetValue=0  RxVelocityTargetValueUnits=deg/s  RxVelocityTargetSpecify=off  RxVelocityTargetPriority=High  RyEquilibriumPosition=0  RyEquilibriumPositionUnits=deg  RySpringStiffness=0  RySpringStiffnessUnits=N*m/deg  RyDampingCoefficient=0  RyDampingCoefficientUnits=N*m/(deg/s)  RyTorqueActuationMode=ComputedTorque  RyMotionActuationMode=InputMotion  RySensePosition=off  RySenseVelocity=off  RySenseAcceleration=off  RySenseTorqueForce=off  RyPositionTargetValue=0  RyPositionTargetValueUnits=deg  RyPositionTargetSpecify=off  RyPositionTargetPriority=High  RyVelocityTargetValue=0  RyVelocityTargetValueUnits=deg/s  RyVelocityTargetSpecify=off  RyVelocityTargetPriority=High  BlockFunction=simmechanics.library.joints.universal_joint
  Right1 : PMIOPort  Port=1  Side=Left
  Right2 : PMIOPort  Port=2  Side=Left
  Right3 : PMIOPort  Port=3  Side=Left
  Left3 : PMIOPort  Port=4  Side=Left
  Left2 : PMIOPort  Port=5  Side=Left
  Left1 : PMIOPort  Port=6  Side=Left
  World : PMIOPort  Port=7  Side=Left
  wires:
  Constant/1 -> Simulink-PS Converter1/1, Simulink-PS Converter3/1
  connections:
  Ball Plane Contact6/LConn1 -- Left1/RConn1
  Ball Plane Contact4/LConn1 -- Left2/RConn1
  Ball Plane Contact3/LConn1 -- Left3/RConn1
  Ball Plane Contact2/LConn1 -- Right3/RConn1
  Ball Plane Contact1/LConn1 -- Right2/RConn1
  Ball Plane Contact5/LConn1 -- Right1/RConn1
  Simulink-PS Converter3/RConn1 -- Universal Joint/LConn2
  Simulink-PS Converter1/RConn1 -- Universal Joint/LConn3
  Plane/RConn1 -- Ball Plane Contact6/RConn1 -- Ball Plane Contact4/RConn1 -- Ball Plane Contact3/RConn1 -- Ball Plane Contact2/RConn1 -- Ball Plane Contact1/RConn1 -- Ball Plane Contact5/RConn1
  Plane/LConn1 -- World/RConn1

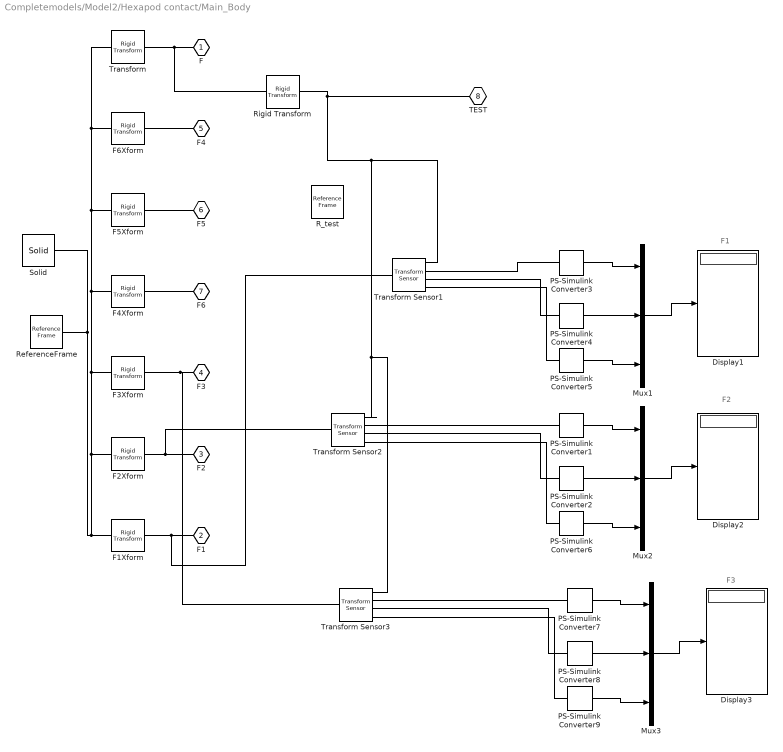
== system Completemodels/Model2/Hexapod contact/Main_Body ==
  note: F3
  note: F2
  note: F1
  Display1 : Display
  Display2 : Display
  Display3 : Display
  F1Xform : sm_lib/Frames and Transforms/Rigid Transform  TranslationMethod=Cartesian  TranslationLengthUnit=mm  TranslationStandardAxis=+Z  TranslationStandardOffset=0  TranslationCartesianOffset=[60.910077554195617 -121.91007755419609 -2.5999999999923125]  TranslationROffset=0  TranslationROffsetUnits=m  TranslationZOffset=0  TranslationZOffsetUnits=m  TranslationThetaOffset=0  TranslationThetaOffsetUnits=deg  RotationMethod=ArbitraryAxis  RotationAngleUnits=rad  RotationStandardAxis=+Z  RotationAngle=2.3561944901923448  RotationArbitraryAxis=[-5.0947287514427085e-14 -3.4119027764489725e-14 -1]  FollAlignAxisA=+X  BaseAlignAxisA=+Y  FollAlignAxisB=+Y  BaseAlignAxisB=+Z  RotationMatrix=[1 0 0; 0 1 0; 0 0 1]  BlockFunction=simmechanics.library.frames_transforms.rigid_transform
  F2Xform : sm_lib/Frames and Transforms/Rigid Transform  TranslationMethod=Cartesian  TranslationLengthUnit=mm  TranslationStandardAxis=+Z  TranslationStandardOffset=0  TranslationCartesianOffset=[103.49999999999983 0 -2.6000000000064678]  TranslationROffset=0  TranslationROffsetUnits=m  TranslationZOffset=0  TranslationZOffsetUnits=m  TranslationThetaOffset=0  TranslationThetaOffsetUnits=deg  RotationMethod=ArbitraryAxis  RotationAngleUnits=rad  RotationStandardAxis=+Z  RotationAngle=1.5707963267948968  RotationArbitraryAxis=[-7.8558330123970482e-14 -1.5711666024794097e-14 -1]  FollAlignAxisA=+X  BaseAlignAxisA=+Y  FollAlignAxisB=+Y  BaseAlignAxisB=+Z  RotationMatrix=[1 0 0; 0 1 0; 0 0 1]  BlockFunction=simmechanics.library.frames_transforms.rigid_transform
  F3Xform : sm_lib/Frames and Transforms/Rigid Transform  TranslationMethod=Cartesian  TranslationLengthUnit=mm  TranslationStandardAxis=+Z  TranslationStandardOffset=0  TranslationCartesianOffset=[60.910077554195631 121.91007755419552 -2.6000000000152843]  TranslationROffset=0  TranslationROffsetUnits=m  TranslationZOffset=0  TranslationZOffsetUnits=m  TranslationThetaOffset=0  TranslationThetaOffsetUnits=deg  RotationMethod=ArbitraryAxis  RotationAngleUnits=rad  RotationStandardAxis=+Z  RotationAngle=0.7853981633974495  RotationArbitraryAxis=[-1.4521728366319145e-13 2.8727636334686562e-14 -1]  FollAlignAxisA=+X  BaseAlignAxisA=+Y  FollAlignAxisB=+Y  BaseAlignAxisB=+Z  RotationMatrix=[1 0 0; 0 1 0; 0 0 1]  BlockFunction=simmechanics.library.frames_transforms.rigid_transform
  F4Xform : sm_lib/Frames and Transforms/Rigid Transform  TranslationMethod=Cartesian  TranslationLengthUnit=mm  TranslationStandardAxis=+Z  TranslationStandardOffset=0  TranslationCartesianOffset=[-60.910077554195958 121.91007755419555 -2.6000000000076282]  TranslationROffset=0  TranslationROffsetUnits=m  TranslationZOffset=0  TranslationZOffsetUnits=m  TranslationThetaOffset=0  TranslationThetaOffsetUnits=deg  RotationMethod=ArbitraryAxis  RotationAngleUnits=rad  RotationStandardAxis=+Z  RotationAngle=0.78539816339744906  RotationArbitraryAxis=[-8.2370619564015128e-14 1.229976324834512e-13 1]  FollAlignAxisA=+X  BaseAlignAxisA=+Y  FollAlignAxisB=+Y  BaseAlignAxisB=+Z  RotationMatrix=[1 0 0; 0 1 0; 0 0 1]  BlockFunction=simmechanics.library.frames_transforms.rigid_transform
  F5Xform : sm_lib/Frames and Transforms/Rigid Transform  TranslationMethod=Cartesian  TranslationLengthUnit=mm  TranslationStandardAxis=+Z  TranslationStandardOffset=0  TranslationCartesianOffset=[-103.50000000000016 0 -2.5999999999934662]  TranslationROffset=0  TranslationROffsetUnits=m  TranslationZOffset=0  TranslationZOffsetUnits=m  TranslationThetaOffset=0  TranslationThetaOffsetUnits=deg  RotationMethod=ArbitraryAxis  RotationAngleUnits=rad  RotationStandardAxis=+Z  RotationAngle=1.5707963267948968  RotationArbitraryAxis=[-1.5711666024794097e-14 7.8558330123970482e-14 1]  FollAlignAxisA=+X  BaseAlignAxisA=+Y  FollAlignAxisB=+Y  BaseAlignAxisB=+Z  RotationMatrix=[1 0 0; 0 1 0; 0 0 1]  BlockFunction=simmechanics.library.frames_transforms.rigid_transform
  F6Xform : sm_lib/Frames and Transforms/Rigid Transform  TranslationMethod=Cartesian  TranslationLengthUnit=mm  TranslationStandardAxis=+Z  TranslationStandardOffset=0  TranslationCartesianOffset=[-60.910077554195937 -121.91007755419606 -2.5999999999846568]  TranslationROffset=0  TranslationROffsetUnits=m  TranslationZOffset=0  TranslationZOffsetUnits=m  TranslationThetaOffset=0  TranslationThetaOffsetUnits=deg  RotationMethod=ArbitraryAxis  RotationAngleUnits=rad  RotationStandardAxis=+Z  RotationAngle=2.3561944901923453  RotationArbitraryAxis=[1.1899376584749339e-14 6.0150968384274875e-14 1]  FollAlignAxisA=+X  BaseAlignAxisA=+Y  FollAlignAxisB=+Y  BaseAlignAxisB=+Z  RotationMatrix=[1 0 0; 0 1 0; 0 0 1]  BlockFunction=simmechanics.library.frames_transforms.rigid_transform
  Mux1 : Mux  Inputs=3
  Mux2 : Mux  Inputs=3
  Mux3 : Mux  Inputs=3
  PS-Simulink Converter{1..9} (9 alike) : nesl_utility/PS-Simulink Converter  PhysicalDomain=network_engine_domain  SubClassName=ps_output  LeftPortType=input  RightPortType=output  PseudoPeriodic=off  Frequencies=[]  Unit=mm  AffineConversion=off
  R_test : sm_lib/Frames and Transforms/Reference Frame  BlockFunction=simmechanics.library.frames_transforms.reference_frame
  ReferenceFrame : sm_lib/Frames and Transforms/Reference Frame  BlockFunction=simmechanics.library.frames_transforms.reference_frame
  Rigid Transform : sm_lib/Frames and Transforms/Rigid Transform  TranslationMethod=None  TranslationLengthUnit=m  TranslationStandardAxis=+Z  TranslationStandardOffset=0  TranslationCartesianOffset=[0 0 0]  TranslationROffset=0  TranslationROffsetUnits=m  TranslationZOffset=0  TranslationZOffsetUnits=m  TranslationThetaOffset=0  TranslationThetaOffsetUnits=deg  RotationMethod=StandardAxis  RotationAngleUnits=deg  RotationStandardAxis=+Z  RotationAngle=-180  RotationArbitraryAxis=[0 0 1]  FollAlignAxisA=+X  BaseAlignAxisA=+Y  FollAlignAxisB=+Y  BaseAlignAxisB=+Z  RotationMatrix=[1 0 0; 0 1 0; 0 0 1]  BlockFunction=simmechanics.library.frames_transforms.rigid_transform
  Solid : sm_lib/Body Elements/Solid  InertiaType=Custom  Mass=0.63100000000000001  MassUnits=kg  CenterOfMass=[2.0291292946603825 -3.6242909829433687 -16.352184508248953]  CenterOfMassUnits=mm  MomentsOfInertia=[273.36575860845227 90.65491799060328 363.95192659905558]  MomentsOfInertiaUnits=kg*mm^2  ProductsOfInertia=[0 0 0]  ProductsOfInertiaUnits=kg*mm^2  DensityBased=on  Density=1000  DensityUnits=kg/(m^3)  GraphicType=FromGeometry  MarkerShape=Sphere  MarkerSize=10  MarkerSizeUnits=m  GraphicVisPropType=SimpleVisualProperties  GraphicDiffuseColor=[0.50196078431372548 0.50196078431372548 0.50196078431372548]  GraphicSpecularColor=[0.5 0.5 0.5 1.0]  GraphicAmbientColor=[0.15 0.15 0.15 1.0]  GraphicEmissiveColor=[0.0 0.0 0.0 1.0]  GraphicShininess=75  GraphicOpacity=1  GeometryShape=FromFile  RectangleSize=[1 1]  RectangleSizeUnits=m  BrickDimensions=[1 1 1]  BrickDimensionUnits=m  CylinderRadius=1  CylinderRadiusUnits=m  CylinderLength=1  CylinderLengthUnits=m  SphereRadius=1  SphereRadiusUnits=m  EllipsoidRadii=[1 1 1]  EllipsoidRadiiUnits=m  ExtrusionCrossSection=[1 1; -1 1; -1 -1; 1 -1]  ExtrusionCrossSectionUnits=m  ExtrusionLength=1  ExtrusionLengthUnits=m  PolygonNumSides=3  PolygonOuterRadius=1  PolygonOuterRadiusUnits=m  ExtGeomFileType=STL  ExtGeomFileName=Main_body_Default_sldprt.STL  ExtGeomFileUnits=mm  RevolutionCrossSection=[1 1; 1 -1; 2 -1; 2 1]  RevolutionCrossSectionUnits=m  RevolutionExtent=Full  RevolutionAngle=180  RevolutionAngleUnits=deg  BlockFunction=simmechanics.library.body_elements.solid
  Transform : sm_lib/Frames and Transforms/Rigid Transform  TranslationMethod=Cartesian  TranslationLengthUnit=mm  TranslationStandardAxis=+Z  TranslationStandardOffset=0  TranslationCartesianOffset=[0 0 0]  TranslationROffset=0  TranslationROffsetUnits=m  TranslationZOffset=0  TranslationZOffsetUnits=m  TranslationThetaOffset=0  TranslationThetaOffsetUnits=deg  RotationMethod=ArbitraryAxis  RotationAngleUnits=rad  RotationStandardAxis=+Z  RotationAngle=0  RotationArbitraryAxis=[0 0 0]  FollAlignAxisA=+X  BaseAlignAxisA=+Y  FollAlignAxisB=+Y  BaseAlignAxisB=+Z  RotationMatrix=[1 0 0; 0 1 0; 0 0 1]  BlockFunction=simmechanics.library.frames_transforms.rigid_transform
  Transform Sensor1 : sm_lib/Frames and Transforms/Transform Sensor  MeasurementFrame=Base  SenseAngle=off  SenseAxis=off  SenseAngle1=off  SenseAngle2=off  SenseAngle3=off  SenseQ=off  SenseR=off  SenseOmegaX=off  SenseOmegaY=off  SenseOmegaZ=off  SenseOmega1=off  SenseOmega2=off  SenseOmega3=off  SenseQDot=off  SenseRDot=off  SenseAlphaX=off  SenseAlphaY=off  SenseAlphaZ=off  SenseAlpha1=off  SenseAlpha2=off  SenseAlpha3=off  SenseQDDot=off  SenseRDDot=off  SenseX=on  SenseY=on  SenseZ=on  SenseRad=off  SenseAzim=off  SenseDist=off  SenseInc=off  SenseXDot=off  SenseYDot=off  SenseZDot=off  SenseRadDot=off  SenseAzimDot=off  SenseDistDot=off  SenseIncDot=off  SenseXDDot=off  SenseYDDot=off  SenseZDDot=off  SenseRadDDot=off  SenseAzimDDot=off  SenseDistDDot=off  SenseIncDDot=off  BlockFunction=simmechanics.library.frames_transforms.transform_sensor
  Transform Sensor2 : sm_lib/Frames and Transforms/Transform Sensor  MeasurementFrame=Base  SenseAngle=off  SenseAxis=off  SenseAngle1=off  SenseAngle2=off  SenseAngle3=off  SenseQ=off  SenseR=off  SenseOmegaX=off  SenseOmegaY=off  SenseOmegaZ=off  SenseOmega1=off  SenseOmega2=off  SenseOmega3=off  SenseQDot=off  SenseRDot=off  SenseAlphaX=off  SenseAlphaY=off  SenseAlphaZ=off  SenseAlpha1=off  SenseAlpha2=off  SenseAlpha3=off  SenseQDDot=off  SenseRDDot=off  SenseX=on  SenseY=on  SenseZ=on  SenseRad=off  SenseAzim=off  SenseDist=off  SenseInc=off  SenseXDot=off  SenseYDot=off  SenseZDot=off  SenseRadDot=off  SenseAzimDot=off  SenseDistDot=off  SenseIncDot=off  SenseXDDot=off  SenseYDDot=off  SenseZDDot=off  SenseRadDDot=off  SenseAzimDDot=off  SenseDistDDot=off  SenseIncDDot=off  BlockFunction=simmechanics.library.frames_transforms.transform_sensor
  Transform Sensor3 : sm_lib/Frames and Transforms/Transform Sensor  MeasurementFrame=Base  SenseAngle=off  SenseAxis=off  SenseAngle1=off  SenseAngle2=off  SenseAngle3=off  SenseQ=off  SenseR=off  SenseOmegaX=off  SenseOmegaY=off  SenseOmegaZ=off  SenseOmega1=off  SenseOmega2=off  SenseOmega3=off  SenseQDot=off  SenseRDot=off  SenseAlphaX=off  SenseAlphaY=off  SenseAlphaZ=off  SenseAlpha1=off  SenseAlpha2=off  SenseAlpha3=off  SenseQDDot=off  SenseRDDot=off  SenseX=on  SenseY=on  SenseZ=on  SenseRad=off  SenseAzim=off  SenseDist=off  SenseInc=off  SenseXDot=off  SenseYDot=off  SenseZDot=off  SenseRadDot=off  SenseAzimDot=off  SenseDistDot=off  SenseIncDot=off  SenseXDDot=off  SenseYDDot=off  SenseZDDot=off  SenseRadDDot=off  SenseAzimDDot=off  SenseDistDDot=off  SenseIncDDot=off  BlockFunction=simmechanics.library.frames_transforms.transform_sensor
  F : PMIOPort  Port=1  Side=Left
  F1 : PMIOPort  Port=2  Side=Left
  F2 : PMIOPort  Port=3  Side=Left
  F3 : PMIOPort  Port=4  Side=Left
  F4 : PMIOPort  Port=5  Side=Right
  F5 : PMIOPort  Port=6  Side=Right
  F6 : PMIOPort  Port=7  Side=Right
  TEST : PMIOPort  Port=8  Side=Right
  wires:
  PS-Simulink Converter7/1 -> Mux3/1
  PS-Simulink Converter8/1 -> Mux3/2
  PS-Simulink Converter9/1 -> Mux3/3
  Mux3/1 -> Display3/1
  PS-Simulink Converter1/1 -> Mux2/1
  PS-Simulink Converter2/1 -> Mux2/2
  PS-Simulink Converter6/1 -> Mux2/3
  Mux2/1 -> Display2/1
  PS-Simulink Converter3/1 -> Mux1/1
  PS-Simulink Converter4/1 -> Mux1/2
  PS-Simulink Converter5/1 -> Mux1/3
  Mux1/1 -> Display1/1
  connections:
  Transform Sensor3/RConn4 -- PS-Simulink Converter9/LConn1
  PS-Simulink Converter7/LConn1 -- Transform Sensor3/RConn2
  PS-Simulink Converter8/LConn1 -- Transform Sensor3/RConn3
  Transform Sensor2/RConn4 -- PS-Simulink Converter6/LConn1
  PS-Simulink Converter2/LConn1 -- Transform Sensor2/RConn3
  PS-Simulink Converter1/LConn1 -- Transform Sensor2/RConn2
  PS-Simulink Converter4/LConn1 -- Transform Sensor1/RConn3
  PS-Simulink Converter3/LConn1 -- Transform Sensor1/RConn2
  Transform Sensor1/RConn4 -- PS-Simulink Converter5/LConn1
  Rigid Transform/RConn1 -- Transform Sensor1/RConn1 -- Transform Sensor3/RConn1 -- Transform Sensor2/RConn1 -- TEST/RConn1
  Transform/RConn1 -- Rigid Transform/LConn1 -- F/RConn1
  F6Xform/RConn1 -- F4/RConn1
  F5Xform/RConn1 -- F5/RConn1
  F4Xform/RConn1 -- F6/RConn1
  F3/RConn1 -- Transform Sensor3/LConn1 -- F3Xform/RConn1
  F2/RConn1 -- Transform Sensor2/LConn1 -- F2Xform/RConn1
  F1/RConn1 -- Transform Sensor1/LConn1 -- F1Xform/RConn1
  ReferenceFrame/RConn1 -- Solid/RConn1 -- F1Xform/LConn1 -- F3Xform/LConn1 -- F4Xform/LConn1 -- F5Xform/LConn1 -- Transform/LConn1 -- F6Xform/LConn1 -- F2Xform/LConn1

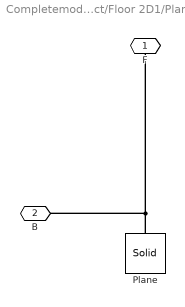
== system Completemodels/Model2/Hexapod contact/Floor 2D1/Plane ==
  Plane : sm_lib/Body Elements/Solid  InertiaType=CalculateFromGeometry  Mass=1  MassUnits=kg  CenterOfMass=[0 0 0]  CenterOfMassUnits=m  MomentsOfInertia=[1 1 1]  MomentsOfInertiaUnits=kg*m^2  ProductsOfInertia=[0 0 0]  ProductsOfInertiaUnits=kg*m^2  DensityBased=on  Density=1000  DensityUnits=kg/(m^3)  GraphicType=FromGeometry  MarkerShape=Sphere  MarkerSize=10  MarkerSizeUnits=m  GraphicVisPropType=SimpleVisualProperties  GraphicDiffuseColor=[0.5 0.5 0.5]  GraphicSpecularColor=[0.5 0.5 0.5 1.0]  GraphicAmbientColor=[0.15 0.15 0.15 1.0]  GraphicEmissiveColor=[0.0 0.0 0.0 1.0]  GraphicShininess=75  GraphicOpacity=1.0  GeometryShape=Brick  RectangleSize=[1 1]  RectangleSizeUnits=m  BrickDimensions=[2.5 2.5 0.05]  BrickDimensionUnits=m  CylinderRadius=1  CylinderRadiusUnits=m  CylinderLength=1  CylinderLengthUnits=m  SphereRadius=1  SphereRadiusUnits=m  EllipsoidRadii=[1 1 1]  EllipsoidRadiiUnits=m  ExtrusionCrossSection=[1 1; -1 1; -1 -1; 1 -1]  ExtrusionCrossSectionUnits=m  ExtrusionLength=1  ExtrusionLengthUnits=m  PolygonNumSides=3  PolygonOuterRadius=1  PolygonOuterRadiusUnits=m  ExtGeomFileType=STL  ExtGeomFileUnits=m  RevolutionCrossSection=[1 1; 1 -1; 2 -1; 2 1]  RevolutionCrossSectionUnits=m  RevolutionExtent=Full  RevolutionAngle=180  RevolutionAngleUnits=deg  BlockFunction=simmechanics.library.body_elements.solid
  F : PMIOPort  Port=1  Side=Right
  B : PMIOPort  Port=2  Side=Left
  connections:
  Plane/RConn1 -- F/RConn1 -- B/RConn1
